simulink subsystem "VCM_main"  (R2021b)
settings: Solver=VariableStepAuto  StartTime=0.0  StopTime=10.0  RelTol=1e-3
undefined symbols (not defined in the file): df, dr, g, gear_f, gear_r, Iwf, Iwr, l, lf, M, Rwf, Rwr
libraries: simulink x47, dspstat3 x2, dspswit3 x1
(part 3 of 4)

== system VCM_main/Error display Box/Error Info3/error memory MC4 ==
  Error info : Inport
  Error triger : Inport  Port=2
  Triggered Subsystem : Subsystem  TreatAsAtomicUnit=on
  error1 : Outport  VectorParamsAs1DForOutWhenUnconnected=off
  error2 : Outport  Port=2  VectorParamsAs1DForOutWhenUnconnected=off
  error3 : Outport  Port=3  VectorParamsAs1DForOutWhenUnconnected=off
  wires:
  Triggered Subsystem/3(Out3) -> error3/1
  Error triger/1 -> Triggered Subsystem/Trigger
  Triggered Subsystem/2(Out2) -> error2/1
  Triggered Subsystem/1(Out1) -> error1/1
  Error info/1 -> Triggered Subsystem/1(In1)

== system VCM_main/VDC/80kw_limitation/Power Limit_last ==
  LimitTorque : Inport
  Power Consumption : Inport  Port=2
  Torque : Inport  Port=3
  Add : Sum  Inputs=+-
  Bus Creator : BusCreator  Inputs=4
  Bus Selector1 : BusSelector  OutputSignals=RR.torque
  Bus Selector2 : BusSelector  OutputSignals=RR,RL,FR,FL
  Bus Selector3 : BusSelector  OutputSignals=FR.torque
  Bus Selector4 : BusSelector  OutputSignals=RR.torque
  Bus Selector5 : BusSelector  OutputSignals=FL.torque
  Compare To Zero : simulink/Logic and Bit Operations/Compare To Zero  relop=<  OutDataTypeStr=boolean
  Constant : Constant  Value=80000
  Divide : Product  Inputs=**
  FeedBack : Subsystem
  FeedBack and Switch : Subsystem
  FeedBack and Switch1 : Subsystem
  FeedBack and Switch2 : Subsystem
  FeedBack and Switch3 : Subsystem
  FeedBack1 : Subsystem
  FeedBack2 : Subsystem
  FeedBack3 : Subsystem
  Gain : Gain  Gain=0
  Scope : Scope
  Scope1 : Scope
  Scope2 : Scope
  TrqOut : Outport  VectorParamsAs1DForOutWhenUnconnected=off
  wires:
  Torque/1 -> Bus Selector4/1, Bus Selector3/1, Bus Selector5/1, Bus Selector1/1
  Bus Selector5/1 -> FeedBack and Switch3/2(Torque)  "<torque>"
  Bus Selector3/1 -> FeedBack and Switch2/2(Torque)  "<torque>"
  Bus Selector1/1 -> FeedBack and Switch1/2(Torque)  "<torque>"
  FeedBack3/1(FB Torque) -> FeedBack and Switch3/1(LimitTorque)
  FeedBack2/1(FB Torque) -> FeedBack and Switch2/1(LimitTorque)
  FeedBack1/1(FB Torque) -> FeedBack and Switch1/1(LimitTorque)
  Bus Selector4/1 -> FeedBack and Switch/2(Torque)  "<torque>"
  FeedBack/1(FB Torque) -> FeedBack and Switch/1(LimitTorque)
  Divide/1 -> FeedBack2/2(FB), FeedBack1/2(FB), FeedBack/2(FB), FeedBack3/2(FB), Scope1/1
  Bus Selector2/4 -> FeedBack3/1(Torque)  "<FL>"
  Bus Selector2/3 -> FeedBack2/1(Torque)  "<FR>"
  Bus Selector2/2 -> FeedBack1/1(Torque)  "<RL>"
  FeedBack and Switch/1(trq) -> Bus Creator/1  "RRtorque"
  FeedBack and Switch3/1(trq) -> Bus Creator/4  "FLtorque"
  Bus Creator/1 -> TrqOut/1, Scope2/1
  FeedBack and Switch1/1(trq) -> Bus Creator/2  "RLtorque"
  FeedBack and Switch2/1(trq) -> Bus Creator/3  "FRtorque"
  Bus Selector2/1 -> FeedBack/1(Torque)  "<RR>"
  LimitTorque/1 -> Bus Selector2/1
  Gain/1 -> Divide/2
  Compare To Zero/1 -> Divide/1
  Add/1 -> Compare To Zero/1, Gain/1
  Power Consumption/1 -> Add/2, Scope/1
  Constant/1 -> Add/1

== system VCM_main/VDC/80kw_limitation/signal select ==
  Torque : Inport
  Bus Creator{,1..3} (4 alike) : BusCreator  Inputs=2
  Bus Creator4 : BusCreator  Inputs=4
  Bus Selector : BusSelector  OutputSignals=RR.torque,RL.torque,FR.torque,FL.torque
  Torque Speed : Outport  VectorParamsAs1DForOutWhenUnconnected=off
  wires:
  Bus Selector/4 -> Bus Creator2/1  "<torque>"
  Bus Selector/3 -> Bus Creator3/1  "<torque>"
  Bus Selector/2 -> Bus Creator1/1  "<torque>"
  Bus Selector/1 -> Bus Creator/1  "<torque>"
  [FL_ActualSpeed] -> Bus Creator2/2  "speed"
  [FR_ActualSpeed] -> Bus Creator3/2  "speed"
  [RL_ActualSpeed] -> Bus Creator1/2  "speed"
  [RR_ActualSpeed] -> Bus Creator/2  "speed"
  Bus Creator4/1 -> Torque Speed/1
  Bus Creator2/1 -> Bus Creator4/4  "FL"
  Bus Creator3/1 -> Bus Creator4/3  "FR"
  Bus Creator1/1 -> Bus Creator4/2  "RL"
  Bus Creator/1 -> Bus Creator4/1  "RR"
  Torque/1 -> Bus Selector/1

== system VCM_main/VDC/DYC1/DYC Switch ==
  Torque In : Inport
  DYC_Torque : Inport  Port=2
  Logical Operator : Logic  AllPortsSameDT=off  OutDataTypeStr=boolean
  Switch : Switch  Criteria=u2 > Threshold  Threshold=0.5
  torque : Outport
  wires:
  Logical Operator/1 -> Switch/2
  [All_bQuitInverterOn] -> Logical Operator/2
  Switch/1 -> torque/1
  [DYCOn] -> Logical Operator/1
  DYC_Torque/1 -> Switch/1  "torque"
  Torque In/1 -> Switch/3

== system VCM_main/VDC/DYC1/DYC Switch1 ==
  Torque In : Inport
  DYC_Torque : Inport  Port=2
  Logical Operator : Logic  AllPortsSameDT=off  OutDataTypeStr=boolean
  Switch : Switch  Criteria=u2 > Threshold  Threshold=0.5
  torque : Outport
  wires:
  Torque In/1 -> Switch/3
  DYC_Torque/1 -> Switch/1  "torque"
  [DYCOn] -> Logical Operator/1
  Switch/1 -> torque/1
  [All_bQuitInverterOn] -> Logical Operator/2
  Logical Operator/1 -> Switch/2

== system VCM_main/VDC/DYC1/DYC Switch2 ==
  Torque In : Inport
  DYC_Torque : Inport  Port=2
  Logical Operator : Logic  AllPortsSameDT=off  OutDataTypeStr=boolean
  Switch : Switch  Criteria=u2 > Threshold  Threshold=0.5
  torque : Outport
  wires:
  Logical Operator/1 -> Switch/2
  [All_bQuitInverterOn] -> Logical Operator/2
  Switch/1 -> torque/1
  [DYCOn] -> Logical Operator/1
  DYC_Torque/1 -> Switch/1  "torque"
  Torque In/1 -> Switch/3

== system VCM_main/VDC/DYC1/DYC Switch3 ==
  Torque In : Inport
  DYC_Torque : Inport  Port=2
  Logical Operator : Logic  AllPortsSameDT=off  OutDataTypeStr=boolean
  Switch : Switch  Criteria=u2 > Threshold  Threshold=0.5
  torque : Outport
  wires:
  Torque In/1 -> Switch/3
  DYC_Torque/1 -> Switch/1  "torque"
  [DYCOn] -> Logical Operator/1
  Switch/1 -> torque/1
  [All_bQuitInverterOn] -> Logical Operator/2
  Logical Operator/1 -> Switch/2

== system VCM_main/VDC/DYC1/DYC main ==
  Total Torque In : Inport
  DriverInput : Inport  Port=2
  Sensor : Inport  Port=3
  Bus Creator : BusCreator  Inputs=6
  Bus Creator1 : BusCreator  Inputs=6
  Bus Creator2 : BusCreator  Inputs=2
  Bus Selector : BusSelector  OutputSignals=Gain,Moment,DYCtrq_RR,DYCtrq_RL,DYCtrq_FR,DYCtrq_FL
  DYC ecopa spec : Subsystem  TreatAsAtomicUnit=on
  DYC mode1 : Subsystem  TreatAsAtomicUnit=on
  If1 : If  IfExpression=u1 == 0  ElseIfExpressions=u1<=1
  Merge : Merge
  Saturation : Saturate  UpperLimit=1  LowerLimit=0
  Terminator : Terminator
  DYC_RR : Outport
  DYC_RL : Outport  Port=2
  DYC_FR : Outport  Port=3
  DYC_FL : Outport  Port=4
  Gain : Outport  Port=5
  Moment : Outport  Port=6
  wires:
  Bus Creator2/1 -> DYC mode1/4(from_steerSW)
  [Kfb2_delta] -> Bus Creator2/2  "Kfb2_delta"
  [Km_delta] -> Bus Creator2/1  "Km_delta"
  [DYCmode] -> Saturation/1
  Bus Selector/6 -> DYC_FL/1  "<DYCtrq_FL>"
  Bus Selector/5 -> DYC_FR/1  "<DYCtrq_FR>"
  Bus Selector/4 -> DYC_RL/1  "<DYCtrq_RL>"
  Bus Selector/3 -> DYC_RR/1  "<DYCtrq_RR>"
  Bus Selector/2 -> Moment/1  "<Moment>"
  Bus Selector/1 -> Gain/1  "<Gain>"
  Merge/1 -> Bus Selector/1
  Bus Creator1/1 -> Merge/2
  Bus Creator/1 -> Merge/1
  DYC mode1/6(DYC_FL) -> Bus Creator1/6
  DYC mode1/5(DYC_FR) -> Bus Creator1/5
  DYC mode1/4(DYC_RL) -> Bus Creator1/4
  DYC mode1/3(DYC_RR) -> Bus Creator1/3
  DYC mode1/2(DYC_M) -> Bus Creator1/2  "Moment"
  DYC mode1/1(DYC_K) -> Bus Creator1/1  "Gain"
  Saturation/1 -> If1/1
  If1/3 -> Terminator/1
  If1/2 -> DYC mode1/Action
  If1/1 -> DYC ecopa spec/Action
  DYC ecopa spec/1(DYC_K) -> Bus Creator/1  "Gain"
  DYC ecopa spec/4(DYC_RL) -> Bus Creator/4
  DYC ecopa spec/5(DYC_FR) -> Bus Creator/5
  DYC ecopa spec/2(DYC_M) -> Bus Creator/2  "Moment"
  DYC ecopa spec/3(DYC_RR) -> Bus Creator/3
  DYC ecopa spec/6(DYC_FL) -> Bus Creator/6
  Total Torque In/1 -> DYC ecopa spec/1(Total Torque In), DYC mode1/1(Total Torque In)
  Sensor/1 -> DYC ecopa spec/3(Sensor), DYC mode1/3(Sensor)
  DriverInput/1 -> DYC ecopa spec/2(DriverInput), DYC mode1/2(DriverInput)

== system VCM_main/VDC/Launch/max rpm ==
  Can Inv : Inport
  Bus Selector4 : BusSelector  OutputSignals=MC_11.MC1_Actual speed value in 1/rpm,MC_31.MC3_Actual speed value in 1/rpm,MC_21.MC2_Actual speed value in 1/rpm,MC_41.MC4_Actual speed value in 1/rpm
  Min : MinMax  Function=max  Inputs=4
  max rpm : Outport
  wires:
  Bus Selector4/2 -> Min/2  "<MC3_Actual speed value in 1/rpm>"
  Bus Selector4/3 -> Min/3  "<MC2_Actual speed value in 1/rpm>"
  Bus Selector4/1 -> Min/1  "<MC1_Actual speed value in 1/rpm>"
  Min/1 -> max rpm/1  "max rpm"
  Can Inv/1 -> Bus Selector4/1
  Bus Selector4/4 -> Min/4  "<MC4_Actual speed value in 1/rpm>"

== system VCM_main/VDC/Subsystem/Subsystem ==
  note: 4コ合計
  In1 : Inport
  IVT : Inport  Port=2
  Bus Selector : BusSelector  OutputSignals=MC_11.MC1_Actual speed value in 1/rpm
  Bus Selector1 : BusSelector  OutputSignals=IVT_Msg_Result_U1
  C : Gain
  Divide : Product  Inputs=**
  Divide1 : Product  Inputs=*//
  Gain : Gain  Gain=100
  Gear : Constant  Value=13.75
  Rated Capacity(A) : Constant  Value=10
  max torque : Outport
  wires:
  Gain/1 -> Divide/2
  Bus Selector1/1 -> Gain/1  "<IVT_Msg_Result_U1>"
  Divide1/1 -> max torque/1  "max torque"
  Gear/1 -> Divide1/3
  IVT/1 -> Bus Selector1/1
  Divide/1 -> Divide1/1
  Bus Selector/1 -> Divide1/2  "<MC1_Actual speed value in 1/rpm>"
  C/1 -> Divide/1
  Rated Capacity(A)/1 -> C/1
  In1/1 -> Bus Selector/1

== system VCM_main/VDC/Subsystem1/Subsystem ==
  CAN from INV : Inport
  IVT : Inport  Port=2
  Bus Selector : BusSelector  OutputSignals=MC_11.MC1_Actual speed value in 1/rpm
  Bus Selector1 : BusSelector  OutputSignals=IVT_Msg_Result_U1
  C : Gain
  Divide : Product  Inputs=**
  Divide1 : Product  Inputs=*//
  Gain : Gain  Gain=100
  Gear : Constant  Value=13.75
  Rated Capacity(A) : Constant  Value=10
  Out1 : Outport
  wires:
  Gain/1 -> Divide/2
  Bus Selector1/1 -> Gain/1  "<IVT_Msg_Result_U1>"
  Divide1/1 -> Out1/1
  Gear/1 -> Divide1/3
  IVT/1 -> Bus Selector1/1
  Divide/1 -> Divide1/1
  Bus Selector/1 -> Divide1/2  "<MC1_Actual speed value in 1/rpm>"
  C/1 -> Divide/1
  Rated Capacity(A)/1 -> C/1
  CAN from INV/1 -> Bus Selector/1

== system VCM_main/VDC/Subsystem1/ideal brake torque for real time ==
  In1 : Inport
  Add : Sum  Inputs=-+
  Add1 : Sum
  Add2 : Sum  Inputs=-+
  Constant5 : Constant
  Divide : Product  Inputs=**
  Divide1 : Product  Inputs=***
  Divide2 : Product  Inputs=*/
  Divide3 : Product  Inputs=**
  Gain : Gain  Gain=0.2
  Gain1 : Gain  Gain=0.2
  Gain2 : Gain  Gain=1/2
  Gain3 : Gain  Gain=1/2
  hight of center of gravity : Constant  Value=0.26
  mass : Constant  Value=280
  static braking balance of front : Constant  Value=0.52
  wheel base : Constant  Value=1.53
  front ideal braking torque : Outport
  rear ideal braking torque : Outport  Port=2
  wires:
  Gain3/1 -> rear ideal braking torque/1
  Gain2/1 -> front ideal braking torque/1
  Gain/1 -> Gain2/1
  Gain1/1 -> Gain3/1
  Add2/1 -> Gain1/1  "rear ideal braking force"
  Add1/1 -> Gain/1  "front ideal braking force"
  In1/1 -> Divide1/1
  Divide/1 -> Add1/1  "front static load"
  Constant5/1 -> Add/2
  hight of center of gravity/1 -> Divide2/1
  Add/1 -> Divide3/2
  wheel base/1 -> Divide2/2
  static braking balance of front/1 -> Add/1, Divide/1
  Divide1/1 -> Add2/1, Add1/2
  Divide3/1 -> Add2/2  "rear static load"
  mass/1 -> Divide1/2, Divide/2, Divide3/1
  Divide2/1 -> Divide1/3

== system VCM_main/VDC/Torque Front//rear distributor Main/Max Torque Limit ==
  note: MAXトルクオーバーしている分だけもう一方に振り直し
  Max Torque : Inport
  torque_front : Inport  Port=2
  torque_rear : Inport  Port=3
  Add10 : Sum  Inputs=-+
  Add11 : Sum
  Add4 : Sum  Inputs=+-
  Add7 : Sum  Inputs=+-
  Add8 : Sum
  Add9 : Sum  Inputs=+-
  Display : Display
  Display5 : Display
  Display6 : Display
  Saturation : Saturate  UpperLimit=inf  LowerLimit=0
  Saturation3 : Saturate  UpperLimit=inf  LowerLimit=0
  torque_front Out : Outport
  torque_rear Out : Outport  Port=2
  wires:
  Max Torque/1 -> Add9/2, Add4/2
  Add11/1 -> torque_rear Out/1
  Add7/1 -> Add11/2
  Add4/1 -> Saturation/1
  Add10/1 -> torque_front Out/1
  Add8/1 -> Add10/2
  torque_rear/1 -> Display6/1, Add7/1, Add4/1
  Add9/1 -> Saturation3/1
  torque_front/1 -> Display5/1, Add8/1, Add9/1
  Saturation3/1 -> Add10/1, Add11/1
  Saturation/1 -> Display/1, Add7/2, Add8/2

== system VCM_main/VDC/Torque Front//rear distributor Main/Min Torque Limit ==
  note: MINトルクオーバーしている分だけもう一方に振り直し
  Min Torque : Inport
  torque_front : Inport  Port=2
  torque_rear : Inport  Port=3
  Add10 : Sum  Inputs=-+
  Add11 : Sum
  Add4 : Sum  Inputs=+-
  Add7 : Sum  Inputs=+-
  Add8 : Sum
  Add9 : Sum  Inputs=+-
  Display{,1..2,5..6} (5 alike) : Display
  Gain : Gain  Gain=-1
  Saturation : Saturate  UpperLimit=0  LowerLimit=-inf
  Saturation3 : Saturate  UpperLimit=0  LowerLimit=-inf
  torque_rear Out : Outport
  torque_front Out : Outport  Port=2
  wires:
  Gain/1 -> Add9/2, Add4/2
  Min Torque/1 -> Gain/1
  Add11/1 -> torque_rear Out/1  "torque_rear"
  Add7/1 -> Add11/2, Display1/1
  Add4/1 -> Saturation/1
  Add10/1 -> torque_front Out/1  "torque_front"
  Add8/1 -> Add10/2
  torque_rear/1 -> Display6/1, Add7/1, Add4/1
  Add9/1 -> Saturation3/1
  torque_front/1 -> Display5/1, Add8/1, Add9/1
  Saturation3/1 -> Add10/1, Add11/1, Display2/1
  Saturation/1 -> Display/1, Add7/2, Add8/2

== system VCM_main/VDC/Torque Front//rear distributor Main/Saturation ==
  u : Inport
  Saturation Dynamic1 : simulink/Discontinuities/Saturation Dynamic  OutMin=[]  OutMax=[]  OutDataTypeStr=Inherit: Same as second input  OutDataType=fixdt(1, 16)  OutScaling=2^-10  DoSatur=off
  y : Outport
  wires:
  [MinTorque] -> Saturation Dynamic1/3
  u/1 -> Saturation Dynamic1/2
  Saturation Dynamic1/1 -> y/1
  [MaxTorque] -> Saturation Dynamic1/1

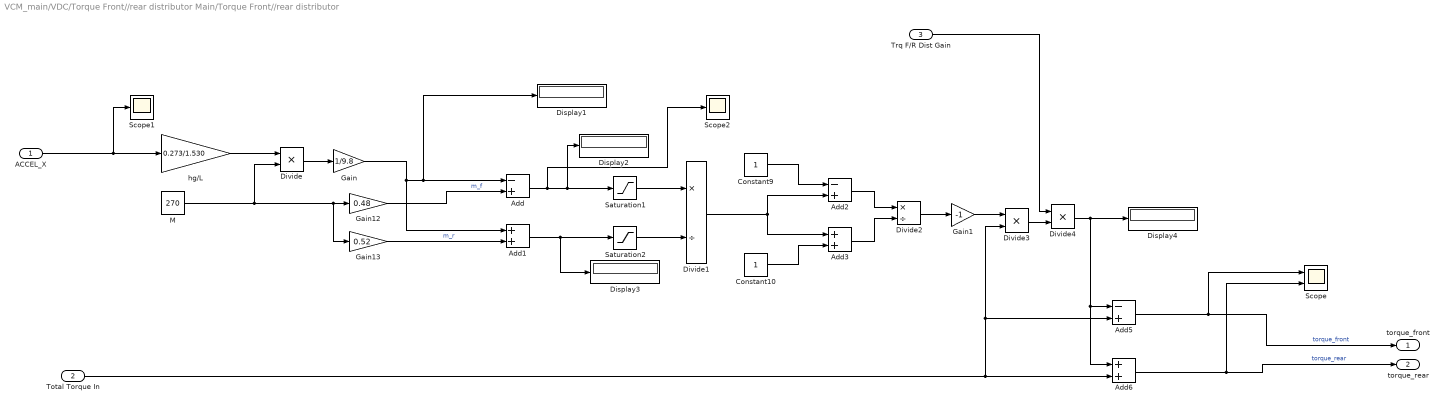
== system VCM_main/VDC/Torque Front//rear distributor Main/Torque Front//rear distributor  ==
  ACCEL_X : Inport
  Total Torque In : Inport  Port=2
  Trq F/R Dist Gain : Inport  Port=3
  Add : Sum  Inputs=-+
  Add1 : Sum
  Add2 : Sum  Inputs=-+
  Add3 : Sum
  Add5 : Sum  Inputs=-+
  Add6 : Sum
  Constant10 : Constant
  Constant9 : Constant
  Display{1..4} (4 alike) : Display
  Divide : Product  Inputs=**
  Divide1 : Product  Inputs=*/
  Divide2 : Product  Inputs=*/
  Divide3 : Product  Inputs=**
  Divide4 : Product  Inputs=**
  Gain : Gain  Gain=1/9.8
  Gain1 : Gain  Gain=-1
  Gain12 : Gain  Gain=0.48
  Gain13 : Gain  Gain=0.52
  M : Constant  Value=270
  Saturation1 : Saturate  UpperLimit=270  LowerLimit=10
  Saturation2 : Saturate  UpperLimit=270  LowerLimit=10
  Scope : Scope  NumInputPorts=2
  Scope1 : Scope
  Scope2 : Scope
  hg/L : Gain  Gain=0.273/1.530
  torque_front : Outport
  torque_rear : Outport  Port=2
  wires:
  Divide/1 -> Gain/1
  Total Torque In/1 -> Divide3/2, Add5/2, Add6/2
  Trq F/R Dist Gain/1 -> Divide4/1
  Divide3/1 -> Divide4/2
  Add5/1 -> torque_front/1, Scope/1  "torque_front"
  Add6/1 -> torque_rear/1, Scope/2  "torque_rear"
  Gain13/1 -> Add1/2  "m_r"
  Saturation1/1 -> Divide1/1
  Add/1 -> Saturation1/1, Display2/1, Scope2/1
  Gain/1 -> Add/1, Display1/1, Add1/1
  Add1/1 -> Saturation2/1, Display3/1
  ACCEL_X/1 -> hg/L/1, Scope1/1
  hg/L/1 -> Divide/1
  Constant10/1 -> Add3/2
  Gain1/1 -> Divide3/1
  Add2/1 -> Divide2/1
  Gain12/1 -> Add/2  "m_f"
  Divide2/1 -> Gain1/1
  Constant9/1 -> Add2/1
  Saturation2/1 -> Divide1/2
  Divide4/1 -> Display4/1, Add5/1, Add6/1
  Add3/1 -> Divide2/2
  Divide1/1 -> Add2/2, Add3/1
  M/1 -> Gain12/1, Gain13/1, Divide/2

== system VCM_main/VDC/Traction Control/Acc Estimater ==
  1/Gear{1..4} (4 alike) : Gain  Gain=gear_r
  Add : Sum  Inputs=++++
  EstLongAcc1 : Scope
  Gain : Gain  Gain=1/(M+2*Iwf/Rwf/Rwf+2*Iwr/Rwr/Rwr)
  Gain1 : Gain  Gain=1/g
  Moving Average : dspstat3/Moving Average  Method=Sliding window  ForgettingFactorPort=off  SpecifyWindowLength=on  WindowLength=10  ForgettingFactor=0.9  SimulateUsing=Code generation
  Rtire{1..4} (4 alike) : Gain  Gain=1/Rwf
  Saturation : Saturate  UpperLimit=1.3*g  LowerLimit=-1.3*g
  EstLongAcc : Outport
  wires:
  [FL_Torque] -> 1/Gear2/1
  Gain/1 -> Moving Average/1  "LongAcc"
  Rtire1/1 -> Add/1
  [RL_Torque] -> 1/Gear4/1
  Rtire3/1 -> Add/3
  1/Gear3/1 -> Rtire4/1
  [FR_Torque] -> 1/Gear1/1
  1/Gear2/1 -> Rtire1/1
  Saturation/1 -> EstLongAcc/1, Gain1/1  "LongAcc"
  Rtire2/1 -> Add/2
  Add/1 -> Gain/1
  1/Gear1/1 -> Rtire2/1
  Gain1/1 -> EstLongAcc1/1
  Rtire4/1 -> Add/4
  1/Gear4/1 -> Rtire3/1
  Moving Average/1 -> Saturation/1
  [RR_Torque] -> 1/Gear3/1

== system VCM_main/VDC/Traction Control/ActualSpeed ==
  Bus Creator : BusCreator  Inputs=4
  ActualSpeed : Outport
  wires:
  [RL_ActualSpeed] -> Bus Creator/3  "RL"
  [FR_ActualSpeed] -> Bus Creator/2  "FR"
  [FL_ActualSpeed] -> Bus Creator/1  "FL"
  [RR_ActualSpeed] -> Bus Creator/4  "RR"
  Bus Creator/1 -> ActualSpeed/1  "ActualSpeed"

== system VCM_main/VDC/Traction Control/Fx Estimater ==
  Bus Creator : BusCreator  Inputs=4
  EstFx : Scope
  FxEstimater : Subsystem
  FxEstimater1 : Subsystem
  FxEstimater2 : Subsystem
  FxEstimater3 : Subsystem
  Fx : Outport
  wires:
  FxEstimater1/1(Fx) -> Bus Creator/2  "FR"
  Bus Creator/1 -> Fx/1, EstFx/1  "Fx"
  FxEstimater3/1(Fx) -> Bus Creator/4  "RR"
  FxEstimater2/1(Fx) -> Bus Creator/3  "RL"
  FxEstimater/1(Fx) -> Bus Creator/1  "FL"
  [FL_Torque] -> FxEstimater/1(Torque)
  [FL_ActualSpeed] -> FxEstimater/2(ActualSpeed)
  [FR_ActualSpeed] -> FxEstimater1/2(ActualSpeed)
  [FR_Torque] -> FxEstimater1/1(Torque)
  [RR_Torque] -> FxEstimater3/1(Torque)
  [RR_ActualSpeed] -> FxEstimater3/2(ActualSpeed)
  [RL_ActualSpeed] -> FxEstimater2/2(ActualSpeed)
  [RL_Torque] -> FxEstimater2/1(Torque)

== system VCM_main/VDC/Traction Control/Load Estimater ==
  Long Acc : Inport
  Sensor : Inport  Port=2
  Steer : Inport  Port=3
  Bus Creator : BusCreator  Inputs=4
  Bus Selector : BusSelector  OutputSignals=CAN_from_IMU_139.VELOCITY_X
  Bus Selector1 : BusSelector  OutputSignals=CAN_from_IMU_121.ACCEL_Y
  Constant : Constant  Value=l
  Divide : Product  Inputs=*/
  Divide1 : Product  Inputs=*/
  EstAcc : Scope  NumInputPorts=2
  EstLoad : Scope
  FR Load Diff : Subsystem  ReferencedSubsystem=FR_Load_Diff
  Gain : Gain  Gain=1/(2*pi)
  Off : Gain  Gain=0
  Product : Product
  RL Load Diff : Subsystem  ReferencedSubsystem=RL_Load_Diff
  Load : Outport
  wires:
  Constant/1 -> Divide/1
  Divide/1 -> Divide1/2  "R"
  RL Load Diff/4 -> Bus Creator/4  "RR"
  Divide1/1 -> EstAcc/2
  Steer/1 -> Gain/1
  RL Load Diff/1 -> Bus Creator/1  "FL"
  FR Load Diff/1 -> RL Load Diff/1  "FrontLoad"
  Bus Selector1/1 -> Off/1  "<ACCEL_Y>"
  FR Load Diff/2 -> RL Load Diff/2  "RearLoad"
  RL Load Diff/2 -> Bus Creator/2  "FR"
  Long Acc/1 -> FR Load Diff/1, EstAcc/1
  RL Load Diff/3 -> Bus Creator/3  "RL"
  Gain/1 -> Divide/2
  Off/1 -> RL Load Diff/3
  Bus Creator/1 -> Load/1, EstLoad/1  "Load"
  Sensor/1 -> Bus Selector1/1, Bus Selector/1
  Bus Selector/1 -> Product/1, Product/2  "<VELOCITY_X>"
  Product/1 -> Divide1/1

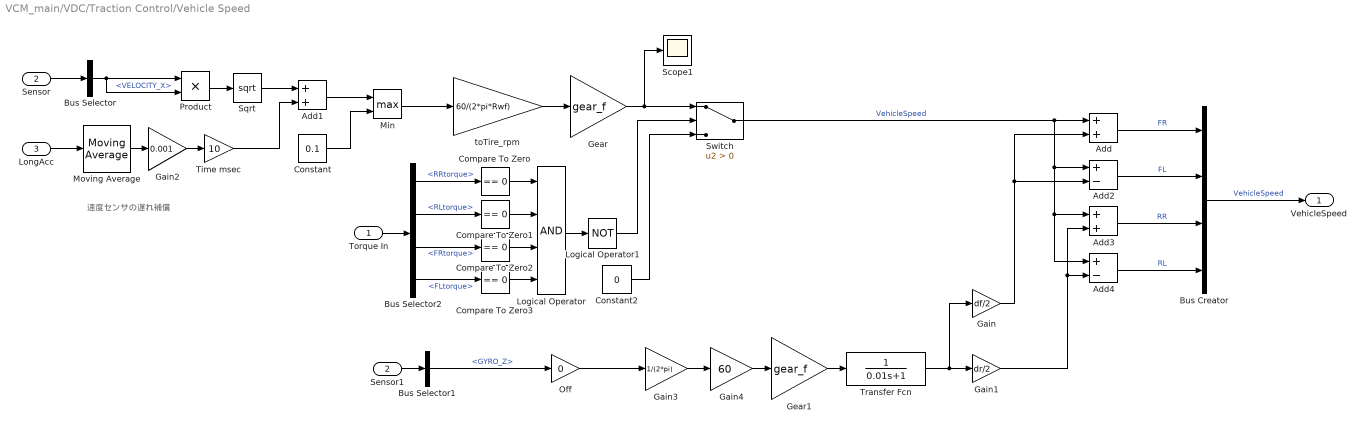
== system VCM_main/VDC/Traction Control/Vehicle Speed ==
  note: 速度センサの遅れ補償
  Torque In : Inport
  Sensor : Inport  Port=2
  LongAcc : Inport  Port=3
  Add : Sum
  Add1 : Sum
  Add2 : Sum  Inputs=+-
  Add3 : Sum
  Add4 : Sum  Inputs=+-
  Bus Creator : BusCreator  Inputs=4
  Bus Selector : BusSelector  OutputSignals=CAN_from_IMU_139.VELOCITY_X
  Bus Selector1 : BusSelector  OutputSignals=CAN_from_IMU_122.GYRO_Z
  Bus Selector2 : BusSelector  OutputSignals=RRtorque,RLtorque,FRtorque,FLtorque
  Compare To Zero{,1..3} (4 alike) : simulink/Logic and Bit Operations/Compare To Zero  relop===  OutDataTypeStr=boolean
  Constant : Constant  Value=0.1
  Constant2 : Constant  Value=0
  Gain : Gain  Gain=df/2
  Gain1 : Gain  Gain=dr/2
  Gain2 : Gain  Gain=0.001
  Gain3 : Gain  Gain=1/(2*pi)
  Gain4 : Gain  Gain=60
  Gear : Gain  Gain=gear_f
  Gear1 : Gain  Gain=gear_f
  Logical Operator : Logic  Inputs=4  AllPortsSameDT=off  OutDataTypeStr=boolean
  Logical Operator1 : Logic  Operator=NOT  AllPortsSameDT=off  OutDataTypeStr=boolean
  Min : MinMax  Function=max  Inputs=2
  Moving Average : dspstat3/Moving Average  Method=Sliding window  ForgettingFactorPort=off  SpecifyWindowLength=on  WindowLength=80  ForgettingFactor=0.9  SimulateUsing=Code generation
  Off : Gain  Gain=0
  Product : Product
  Scope1 : Scope
  Sensor1 : InportShadow  Port=2
  Sqrt : Sqrt  SaturateOnIntegerOverflow=on
  Switch : Switch  Criteria=u2 > Threshold
  Time msec : Gain  Gain=10
  Transfer Fcn : TransferFcn  Denominator=[0.01 1]
  toTire_rpm : Gain  Gain=60/(2*pi*Rwf)
  VehicleSpeed : Outport
  wires:
  Gain3/1 -> Gain4/1
  Bus Selector1/1 -> Off/1  "<GYRO_Z>"
  Product/1 -> Sqrt/1
  Transfer Fcn/1 -> Gain1/1, Gain/1
  Bus Selector/1 -> Product/1, Product/2  "<VELOCITY_X>"
  Switch/1 -> Add/1, Add2/1, Add4/1, Add3/1  "VehicleSpeed"
  Compare To Zero/1 -> Logical Operator/1
  Sensor/1 -> Bus Selector/1
  Bus Selector2/4 -> Compare To Zero3/1  "<FLtorque>"
  Compare To Zero2/1 -> Logical Operator/3
  Torque In/1 -> Bus Selector2/1
  LongAcc/1 -> Moving Average/1
  Sqrt/1 -> Add1/1
  Gear/1 -> Scope1/1, Switch/1
  toTire_rpm/1 -> Gear/1
  Gain1/1 -> Add3/2, Add4/2
  Logical Operator/1 -> Logical Operator1/1
  Add3/1 -> Bus Creator/3  "RR"
  Bus Selector2/1 -> Compare To Zero/1  "<RRtorque>"
  Logical Operator1/1 -> Switch/2
  Sensor1/1 -> Bus Selector1/1
  Compare To Zero3/1 -> Logical Operator/4
  Constant/1 -> Min/2
  Bus Selector2/2 -> Compare To Zero1/1  "<RLtorque>"
  Time msec/1 -> Add1/2
  Bus Selector2/3 -> Compare To Zero2/1  "<FRtorque>"
  Compare To Zero1/1 -> Logical Operator/2
  Off/1 -> Gain3/1
  Constant2/1 -> Switch/3
  Min/1 -> toTire_rpm/1
  Gain/1 -> Add/2, Add2/2
  Add1/1 -> Min/1
  Add2/1 -> Bus Creator/2  "FL"
  Moving Average/1 -> Gain2/1
  Add/1 -> Bus Creator/1  "FR"
  Add4/1 -> Bus Creator/4  "RL"
  Gain2/1 -> Time msec/1
  Gain4/1 -> Gear1/1
  Bus Creator/1 -> VehicleSpeed/1  "VehicleSpeed"
  Gear1/1 -> Transfer Fcn/1

== system VCM_main/VDC/VCM_Status/Sliprate ==
  from Sensor : Inport
  Bus Creator : BusCreator  Inputs=4
  Bus Selector4 : BusSelector  OutputSignals=CAN_from_IMU_139.VELOCITY_X
  Scope : Scope  NumInputPorts=4
  SlipRateClc FL : Subsystem  ReferencedSubsystem=SlipRateClc
  SlipRateClc FR : Subsystem  ReferencedSubsystem=SlipRateClc
  SlipRateClc RL : Subsystem  ReferencedSubsystem=SlipRateClc
  SlipRateClc RR : Subsystem  ReferencedSubsystem=SlipRateClc
  Tire rpm{,1..3} (4 alike) : Gain  Gain=1/gear_f
  to m/s{,1..3} (4 alike) : Gain  Gain=(2*pi*Rwf)/60
  Sliprate : Outport
  wires:
  to m/s1/1 -> SlipRateClc RR/1
  Tire rpm3/1 -> to m/s3/1
  SlipRateClc FR/1 -> Bus Creator/4, Scope/4  "FR"
  Bus Selector4/1 -> SlipRateClc FR/2, SlipRateClc RL/2, SlipRateClc RR/2, SlipRateClc FL/2  "<VELOCITY_X>"
  SlipRateClc RR/1 -> Bus Creator/2, Scope/2  "RR"
  SlipRateClc FL/1 -> Bus Creator/1, Scope/1  "FL"
  Bus Creator/1 -> Sliprate/1  "Sliprate"
  SlipRateClc RL/1 -> Bus Creator/3, Scope/3  "RL"
  Tire rpm1/1 -> to m/s1/1
  to m/s/1 -> SlipRateClc FL/1
  [FL_ActualSpeed] -> Tire rpm/1
  to m/s2/1 -> SlipRateClc RL/1
  Tire rpm/1 -> to m/s/1
  [RL_ActualSpeed] -> Tire rpm2/1
  [FR_ActualSpeed] -> Tire rpm3/1
  [RR_ActualSpeed] -> Tire rpm1/1
  to m/s3/1 -> SlipRateClc FR/1
  Tire rpm2/1 -> to m/s2/1
  from Sensor/1 -> Bus Selector4/1

== system VCM_main/VDC/VCM_Status/VCMStatus_bus ==
  In1 : Inport
  Bus Creator1 : BusCreator  Inputs=7
  Logical Operator1 : Logic  AllPortsSameDT=off  OutDataTypeStr=boolean
  VCMStatus : Outport
  wires:
  Bus Creator1/1 -> VCMStatus/1  "VCMStatus"
  In1/1 -> Logical Operator1/1
  [PowerLimitOn] -> Bus Creator1/7  "80kWOn"
  [TCOn] -> Bus Creator1/4  "TCOn"
  Logical Operator1/1 -> Bus Creator1/1  "VDCStatus"
  [VDCOn] -> Logical Operator1/2
  [DYCOn] -> Bus Creator1/6  "DYCOn"
  [ABSOn] -> Bus Creator1/5  "ABSOn"
  [BrakeOverRide] -> Bus Creator1/3  "BrakeOverRide"
  [APPS_SafetyError] -> Bus Creator1/2  "APPS_SafetyError"

== system VCM_main/Error display Box/Error Info/error memory MC1/Triggered Subsystem ==
  In1 : Inport
  Trigger : TriggerPort  VariantControl=Variant
  Delay : Delay  DelayLength=1  InitialCondition=0
  Delay1 : Delay  InitialCondition=0
  Out1 : Outport  VectorParamsAs1DForOutWhenUnconnected=off
  Out2 : Outport  Port=2  InitialOutput=[0]  VectorParamsAs1DForOutWhenUnconnected=off
  Out3 : Outport  Port=3  InitialOutput=[0]  VectorParamsAs1DForOutWhenUnconnected=off
  wires:
  Delay1/1 -> Out3/1
  Delay/1 -> Out2/1
  In1/1 -> Out1/1, Delay1/1, Delay/1

== system VCM_main/Error display Box/Error Info/error memory MC2/Triggered Subsystem ==
  In1 : Inport
  Trigger : TriggerPort  VariantControl=Variant
  Delay : Delay  DelayLength=1  InitialCondition=0
  Delay1 : Delay  InitialCondition=0
  Out1 : Outport  VectorParamsAs1DForOutWhenUnconnected=off
  Out2 : Outport  Port=2  InitialOutput=[0]  VectorParamsAs1DForOutWhenUnconnected=off
  Out3 : Outport  Port=3  InitialOutput=[0]  VectorParamsAs1DForOutWhenUnconnected=off
  wires:
  Delay1/1 -> Out3/1
  Delay/1 -> Out2/1
  In1/1 -> Out1/1, Delay1/1, Delay/1

== system VCM_main/Error display Box/Error Info/error memory MC3/Triggered Subsystem ==
  In1 : Inport
  Trigger : TriggerPort  VariantControl=Variant
  Delay : Delay  DelayLength=1  InitialCondition=0
  Delay1 : Delay  InitialCondition=0
  Out1 : Outport  VectorParamsAs1DForOutWhenUnconnected=off
  Out2 : Outport  Port=2  InitialOutput=[0]  VectorParamsAs1DForOutWhenUnconnected=off
  Out3 : Outport  Port=3  InitialOutput=[0]  VectorParamsAs1DForOutWhenUnconnected=off
  wires:
  Delay1/1 -> Out3/1
  Delay/1 -> Out2/1
  In1/1 -> Out1/1, Delay1/1, Delay/1

== system VCM_main/Error display Box/Error Info/error memory MC4/Triggered Subsystem ==
  In1 : Inport
  Trigger : TriggerPort  VariantControl=Variant
  Delay : Delay  DelayLength=1  InitialCondition=0
  Delay1 : Delay  InitialCondition=0
  Out1 : Outport  VectorParamsAs1DForOutWhenUnconnected=off
  Out2 : Outport  Port=2  InitialOutput=[0]  VectorParamsAs1DForOutWhenUnconnected=off
  Out3 : Outport  Port=3  InitialOutput=[0]  VectorParamsAs1DForOutWhenUnconnected=off
  wires:
  Delay1/1 -> Out3/1
  Delay/1 -> Out2/1
  In1/1 -> Out1/1, Delay1/1, Delay/1

== system VCM_main/Error display Box/Error Info1/error memory MC1/Triggered Subsystem ==
  In1 : Inport
  Trigger : TriggerPort  VariantControl=Variant
  Delay : Delay  DelayLength=1  InitialCondition=0
  Delay1 : Delay  InitialCondition=0
  Out1 : Outport  VectorParamsAs1DForOutWhenUnconnected=off
  Out2 : Outport  Port=2  InitialOutput=[0]  VectorParamsAs1DForOutWhenUnconnected=off
  Out3 : Outport  Port=3  InitialOutput=[0]  VectorParamsAs1DForOutWhenUnconnected=off
  wires:
  Delay1/1 -> Out3/1
  Delay/1 -> Out2/1
  In1/1 -> Out1/1, Delay/1, Delay1/1

== system VCM_main/Error display Box/Error Info1/error memory MC2/Triggered Subsystem ==
  In1 : Inport
  Trigger : TriggerPort  VariantControl=Variant
  Delay : Delay  DelayLength=1  InitialCondition=0
  Delay1 : Delay  InitialCondition=0
  Out1 : Outport  VectorParamsAs1DForOutWhenUnconnected=off
  Out2 : Outport  Port=2  InitialOutput=[0]  VectorParamsAs1DForOutWhenUnconnected=off
  Out3 : Outport  Port=3  InitialOutput=[0]  VectorParamsAs1DForOutWhenUnconnected=off
  wires:
  Delay1/1 -> Out3/1
  Delay/1 -> Out2/1
  In1/1 -> Out1/1, Delay/1, Delay1/1

== system VCM_main/Error display Box/Error Info1/error memory MC3/Triggered Subsystem ==
  In1 : Inport
  Trigger : TriggerPort  VariantControl=Variant
  Delay : Delay  DelayLength=1  InitialCondition=0
  Delay1 : Delay  InitialCondition=0
  Out1 : Outport  VectorParamsAs1DForOutWhenUnconnected=off
  Out2 : Outport  Port=2  InitialOutput=[0]  VectorParamsAs1DForOutWhenUnconnected=off
  Out3 : Outport  Port=3  InitialOutput=[0]  VectorParamsAs1DForOutWhenUnconnected=off
  wires:
  Delay1/1 -> Out3/1
  Delay/1 -> Out2/1
  In1/1 -> Out1/1, Delay/1, Delay1/1

== system VCM_main/Error display Box/Error Info1/error memory MC4/Triggered Subsystem ==
  In1 : Inport
  Trigger : TriggerPort  VariantControl=Variant
  Delay : Delay  DelayLength=1  InitialCondition=0
  Delay1 : Delay  InitialCondition=0
  Out1 : Outport  VectorParamsAs1DForOutWhenUnconnected=off
  Out2 : Outport  Port=2  InitialOutput=[0]  VectorParamsAs1DForOutWhenUnconnected=off
  Out3 : Outport  Port=3  InitialOutput=[0]  VectorParamsAs1DForOutWhenUnconnected=off
  wires:
  Delay1/1 -> Out3/1
  Delay/1 -> Out2/1
  In1/1 -> Out1/1, Delay/1, Delay1/1

== system VCM_main/Error display Box/Error Info2/error memory MC1/Triggered Subsystem ==
  In1 : Inport
  Trigger : TriggerPort  VariantControl=Variant
  Delay : Delay  DelayLength=1  InitialCondition=0
  Delay1 : Delay  InitialCondition=0
  Out1 : Outport  VectorParamsAs1DForOutWhenUnconnected=off
  Out2 : Outport  Port=2  InitialOutput=[0]  VectorParamsAs1DForOutWhenUnconnected=off
  Out3 : Outport  Port=3  InitialOutput=[0]  VectorParamsAs1DForOutWhenUnconnected=off
  wires:
  Delay1/1 -> Out3/1
  Delay/1 -> Out2/1
  In1/1 -> Out1/1, Delay/1, Delay1/1

== system VCM_main/Error display Box/Error Info2/error memory MC2/Triggered Subsystem ==
  In1 : Inport
  Trigger : TriggerPort  VariantControl=Variant
  Delay : Delay  DelayLength=1  InitialCondition=0
  Delay1 : Delay  InitialCondition=0
  Out1 : Outport  VectorParamsAs1DForOutWhenUnconnected=off
  Out2 : Outport  Port=2  InitialOutput=[0]  VectorParamsAs1DForOutWhenUnconnected=off
  Out3 : Outport  Port=3  InitialOutput=[0]  VectorParamsAs1DForOutWhenUnconnected=off
  wires:
  Delay1/1 -> Out3/1
  Delay/1 -> Out2/1
  In1/1 -> Out1/1, Delay/1, Delay1/1

== system VCM_main/Error display Box/Error Info2/error memory MC3/Triggered Subsystem ==
  In1 : Inport
  Trigger : TriggerPort  VariantControl=Variant
  Delay : Delay  DelayLength=1  InitialCondition=0
  Delay1 : Delay  InitialCondition=0
  Out1 : Outport  VectorParamsAs1DForOutWhenUnconnected=off
  Out2 : Outport  Port=2  InitialOutput=[0]  VectorParamsAs1DForOutWhenUnconnected=off
  Out3 : Outport  Port=3  InitialOutput=[0]  VectorParamsAs1DForOutWhenUnconnected=off
  wires:
  Delay1/1 -> Out3/1
  Delay/1 -> Out2/1
  In1/1 -> Out1/1, Delay/1, Delay1/1

== system VCM_main/Error display Box/Error Info2/error memory MC4/Triggered Subsystem ==
  In1 : Inport
  Trigger : TriggerPort  VariantControl=Variant
  Delay : Delay  DelayLength=1  InitialCondition=0
  Delay1 : Delay  InitialCondition=0
  Out1 : Outport  VectorParamsAs1DForOutWhenUnconnected=off
  Out2 : Outport  Port=2  InitialOutput=[0]  VectorParamsAs1DForOutWhenUnconnected=off
  Out3 : Outport  Port=3  InitialOutput=[0]  VectorParamsAs1DForOutWhenUnconnected=off
  wires:
  Delay1/1 -> Out3/1
  Delay/1 -> Out2/1
  In1/1 -> Out1/1, Delay/1, Delay1/1

== system VCM_main/Error display Box/Error Info3/error memory MC1/Triggered Subsystem ==
  In1 : Inport
  Trigger : TriggerPort  VariantControl=Variant
  Delay : Delay  DelayLength=1  InitialCondition=0
  Delay1 : Delay  InitialCondition=0
  Out1 : Outport  VectorParamsAs1DForOutWhenUnconnected=off
  Out2 : Outport  Port=2  InitialOutput=[0]  VectorParamsAs1DForOutWhenUnconnected=off
  Out3 : Outport  Port=3  InitialOutput=[0]  VectorParamsAs1DForOutWhenUnconnected=off
  wires:
  Delay1/1 -> Out3/1
  Delay/1 -> Out2/1
  In1/1 -> Out1/1, Delay/1, Delay1/1

== system VCM_main/Error display Box/Error Info3/error memory MC2/Triggered Subsystem ==
  In1 : Inport
  Trigger : TriggerPort  VariantControl=Variant
  Delay : Delay  DelayLength=1  InitialCondition=0
  Delay1 : Delay  InitialCondition=0
  Out1 : Outport  VectorParamsAs1DForOutWhenUnconnected=off
  Out2 : Outport  Port=2  InitialOutput=[0]  VectorParamsAs1DForOutWhenUnconnected=off
  Out3 : Outport  Port=3  InitialOutput=[0]  VectorParamsAs1DForOutWhenUnconnected=off
  wires:
  Delay1/1 -> Out3/1
  Delay/1 -> Out2/1
  In1/1 -> Out1/1, Delay/1, Delay1/1

== system VCM_main/Error display Box/Error Info3/error memory MC3/Triggered Subsystem ==
  In1 : Inport
  Trigger : TriggerPort  VariantControl=Variant
  Delay : Delay  DelayLength=1  InitialCondition=0
  Delay1 : Delay  InitialCondition=0
  Out1 : Outport  VectorParamsAs1DForOutWhenUnconnected=off
  Out2 : Outport  Port=2  InitialOutput=[0]  VectorParamsAs1DForOutWhenUnconnected=off
  Out3 : Outport  Port=3  InitialOutput=[0]  VectorParamsAs1DForOutWhenUnconnected=off
  wires:
  Delay1/1 -> Out3/1
  Delay/1 -> Out2/1
  In1/1 -> Out1/1, Delay/1, Delay1/1

== system VCM_main/Error display Box/Error Info3/error memory MC4/Triggered Subsystem ==
  In1 : Inport
  Trigger : TriggerPort  VariantControl=Variant
  Delay : Delay  DelayLength=1  InitialCondition=0
  Delay1 : Delay  InitialCondition=0
  Out1 : Outport  VectorParamsAs1DForOutWhenUnconnected=off
  Out2 : Outport  Port=2  InitialOutput=[0]  VectorParamsAs1DForOutWhenUnconnected=off
  Out3 : Outport  Port=3  InitialOutput=[0]  VectorParamsAs1DForOutWhenUnconnected=off
  wires:
  Delay1/1 -> Out3/1
  Delay/1 -> Out2/1
  In1/1 -> Out1/1, Delay/1, Delay1/1

== system VCM_main/VDC/80kw_limitation/Power Limit_last/FeedBack ==
  Torque : Inport
  FB : Inport  Port=2
  Add : Sum
  Bus Selector3 : BusSelector  OutputSignals=torque
  FB Torque : Outport
  wires:
  Torque/1 -> Bus Selector3/1
  Add/1 -> FB Torque/1
  FB/1 -> Add/2
  Bus Selector3/1 -> Add/1  "<torque>"

== system VCM_main/VDC/80kw_limitation/Power Limit_last/FeedBack and Switch ==
  LimitTorque : Inport
  Torque : Inport  Port=2
  Max : MinMax  Function=max  Inputs=2
  Min : MinMax  Inputs=2
  Saturation Dynamic : simulink/Discontinuities/Saturation Dynamic  OutMin=[]  OutMax=[]  OutDataTypeStr=Inherit: Same as second input  OutDataType=fixdt(1, 16)  OutScaling=2^-10  DoSatur=off
  Switch : Switch  Criteria=u2 > Threshold
  Switch1 : Switch  Criteria=u2 > Threshold
  trq : Outport
  wires:
  [MinTorque] -> Saturation Dynamic/3
  Saturation Dynamic/1 -> trq/1
  Switch1/1 -> Saturation Dynamic/1  "torque"
  [PowerLimitOn] -> Switch1/2
  Switch/1 -> Switch1/1  "torque"
  Min/1 -> Switch/1
  Max/1 -> Switch/3
  Torque/1 -> Min/1, Switch/2, Max/2, Switch1/3, Saturation Dynamic/2
  LimitTorque/1 -> Min/2, Max/1

== system VCM_main/VDC/80kw_limitation/Power Limit_last/FeedBack and Switch1 ==
  LimitTorque : Inport
  Torque : Inport  Port=2
  Max : MinMax  Function=max  Inputs=2
  Min : MinMax  Inputs=2
  Saturation Dynamic : simulink/Discontinuities/Saturation Dynamic  OutMin=[]  OutMax=[]  OutDataTypeStr=Inherit: Same as second input  OutDataType=fixdt(1, 16)  OutScaling=2^-10  DoSatur=off
  Switch : Switch  Criteria=u2 > Threshold
  Switch1 : Switch  Criteria=u2 > Threshold
  trq : Outport
  wires:
  LimitTorque/1 -> Max/1, Min/2
  Torque/1 -> Saturation Dynamic/2, Switch1/3, Max/2, Switch/2, Min/1
  Max/1 -> Switch/3
  Min/1 -> Switch/1
  Switch/1 -> Switch1/1  "torque"
  [PowerLimitOn] -> Switch1/2
  Switch1/1 -> Saturation Dynamic/1  "torque"
  Saturation Dynamic/1 -> trq/1
  [MinTorque] -> Saturation Dynamic/3

== system VCM_main/VDC/80kw_limitation/Power Limit_last/FeedBack and Switch2 ==
  LimitTorque : Inport
  Torque : Inport  Port=2
  Max : MinMax  Function=max  Inputs=2
  Min : MinMax  Inputs=2
  Saturation Dynamic : simulink/Discontinuities/Saturation Dynamic  OutMin=[]  OutMax=[]  OutDataTypeStr=Inherit: Same as second input  OutDataType=fixdt(1, 16)  OutScaling=2^-10  DoSatur=off
  Switch : Switch  Criteria=u2 > Threshold
  Switch1 : Switch  Criteria=u2 > Threshold
  trq : Outport
  wires:
  [MinTorque] -> Saturation Dynamic/3
  Saturation Dynamic/1 -> trq/1
  Switch1/1 -> Saturation Dynamic/1  "torque"
  [PowerLimitOn] -> Switch1/2
  Switch/1 -> Switch1/1  "torque"
  Min/1 -> Switch/1
  Max/1 -> Switch/3
  Torque/1 -> Min/1, Switch/2, Max/2, Switch1/3, Saturation Dynamic/2
  LimitTorque/1 -> Min/2, Max/1

== system VCM_main/VDC/80kw_limitation/Power Limit_last/FeedBack and Switch3 ==
  LimitTorque : Inport
  Torque : Inport  Port=2
  Max : MinMax  Function=max  Inputs=2
  Min : MinMax  Inputs=2
  Saturation Dynamic : simulink/Discontinuities/Saturation Dynamic  OutMin=[]  OutMax=[]  OutDataTypeStr=Inherit: Same as second input  OutDataType=fixdt(1, 16)  OutScaling=2^-10  DoSatur=off
  Switch : Switch  Criteria=u2 > Threshold
  Switch1 : Switch  Criteria=u2 > Threshold
  trq : Outport
  wires:
  LimitTorque/1 -> Max/1, Min/2
  Torque/1 -> Saturation Dynamic/2, Switch1/3, Max/2, Switch/2, Min/1
  Max/1 -> Switch/3
  Min/1 -> Switch/1
  Switch/1 -> Switch1/1  "torque"
  [PowerLimitOn] -> Switch1/2
  Switch1/1 -> Saturation Dynamic/1  "torque"
  Saturation Dynamic/1 -> trq/1
  [MinTorque] -> Saturation Dynamic/3

== system VCM_main/VDC/80kw_limitation/Power Limit_last/FeedBack1 ==
  Torque : Inport
  FB : Inport  Port=2
  Add : Sum
  Bus Selector3 : BusSelector  OutputSignals=torque
  FB Torque : Outport
  wires:
  Bus Selector3/1 -> Add/1  "<torque>"
  FB/1 -> Add/2
  Add/1 -> FB Torque/1
  Torque/1 -> Bus Selector3/1

== system VCM_main/VDC/80kw_limitation/Power Limit_last/FeedBack2 ==
  Torque : Inport
  FB : Inport  Port=2
  Add : Sum
  Bus Selector3 : BusSelector  OutputSignals=torque
  FB Torque : Outport
  wires:
  Torque/1 -> Bus Selector3/1
  Add/1 -> FB Torque/1
  FB/1 -> Add/2
  Bus Selector3/1 -> Add/1  "<torque>"

== system VCM_main/VDC/80kw_limitation/Power Limit_last/FeedBack3 ==
  Torque : Inport
  FB : Inport  Port=2
  Add : Sum
  Bus Selector3 : BusSelector  OutputSignals=torque
  FB Torque : Outport
  wires:
  Bus Selector3/1 -> Add/1  "<torque>"
  FB/1 -> Add/2
  Add/1 -> FB Torque/1
  Torque/1 -> Bus Selector3/1

== system VCM_main/VDC/DYC1/DYC main/DYC ecopa spec ==
  Total Torque In : Inport
  DriverInput : Inport  Port=2
  Sensor : Inport  Port=3
  Action Port : ActionPort
  DYC mode2 : Subsystem
  DYC_K : Outport
  DYC_M : Outport  Port=2
  DYC_RR : Outport  Port=3
  DYC_RL : Outport  Port=4
  DYC_FR : Outport  Port=5
  DYC_FL : Outport  Port=6
  wires:
  DYC mode2/6(DYC_FL) -> DYC_FL/1
  DYC mode2/5(DYC_FR) -> DYC_FR/1
  DYC mode2/4(DYC_RL) -> DYC_RL/1
  DYC mode2/3(DYC_RR) -> DYC_RR/1
  DYC mode2/2(DYC_M) -> DYC_M/1  "Moment"
  Sensor/1 -> DYC mode2/3(Sensor)
  DriverInput/1 -> DYC mode2/2(DriverInput)
  DYC mode2/1(DYC_K) -> DYC_K/1  "Gain"
  Total Torque In/1 -> DYC mode2/1(Total Torque In)

== system VCM_main/VDC/DYC1/DYC main/DYC mode1 ==
  Total Torque In : Inport
  DriverInput : Inport  Port=2
  Sensor : Inport  Port=3
  from_steerSW : Inport  Port=4
  Action Port : ActionPort
  DYC mode1 : Subsystem
  DYC_K : Outport
  DYC_M : Outport  Port=2
  DYC_RR : Outport  Port=3
  DYC_RL : Outport  Port=4
  DYC_FR : Outport  Port=5
  DYC_FL : Outport  Port=6
  wires:
  from_steerSW/1 -> DYC mode1/4(from_steerswitch)
  DYC mode1/6(DYC_FL) -> DYC_FL/1
  DYC mode1/5(DYC_FR) -> DYC_FR/1
  DYC mode1/4(DYC_RL) -> DYC_RL/1
  DYC mode1/3(DYC_RR) -> DYC_RR/1
  DYC mode1/2(DYC_M) -> DYC_M/1  "Moment"
  Sensor/1 -> DYC mode1/3(Sensor)
  DriverInput/1 -> DYC mode1/2(DriverInput)
  DYC mode1/1(DYC_K) -> DYC_K/1  "Gain"
  Total Torque In/1 -> DYC mode1/1(Total Torque In)

== system VCM_main/VDC/Traction Control/Fx Estimater/FxEstimater ==
  Torque : Inport
  ActualSpeed : Inport  Port=2
  Add4 : Sum  Inputs=+-
  Discrete Derivative : simulink/Discrete/Discrete Derivative  gainval=1.0  ICPrevScaledInput=0.0  OutMin=[]  OutMax=[]  OutDataType=fixdt(1, 16)  OutScaling=2^-10  DoSatur=off
  Gain : Gain  Gain=gear_f
  Gain1 : Gain  Gain=1/60
  Gain2 : Gain  Gain=2*pi
  Gain3 : Gain  Gain=1/gear_f
  Gain4 : Gain  Gain=Iwf
  Gain5 : Gain  Gain=1/Rwf
  Fx : Outport
  wires:
  Gain1/1 -> Gain2/1
  Gain2/1 -> Discrete Derivative/1
  Torque/1 -> Gain/1
  Discrete Derivative/1 -> Gain4/1
  Gain/1 -> Add4/1
  Add4/1 -> Gain5/1
  Gain5/1 -> Fx/1
  Gain4/1 -> Add4/2
  ActualSpeed/1 -> Gain3/1
  Gain3/1 -> Gain1/1

== system VCM_main/VDC/Traction Control/Fx Estimater/FxEstimater1 ==
  Torque : Inport
  ActualSpeed : Inport  Port=2
  Add4 : Sum  Inputs=+-
  Discrete Derivative : simulink/Discrete/Discrete Derivative  gainval=1.0  ICPrevScaledInput=0.0  OutMin=[]  OutMax=[]  OutDataType=fixdt(1, 16)  OutScaling=2^-10  DoSatur=off
  Gain : Gain  Gain=gear_f
  Gain1 : Gain  Gain=1/60
  Gain2 : Gain  Gain=2*pi
  Gain3 : Gain  Gain=1/gear_f
  Gain4 : Gain  Gain=Iwf
  Gain5 : Gain  Gain=1/Rwf
  Fx : Outport
  wires:
  Gain3/1 -> Gain1/1
  ActualSpeed/1 -> Gain3/1
  Gain4/1 -> Add4/2
  Gain5/1 -> Fx/1
  Add4/1 -> Gain5/1
  Gain/1 -> Add4/1
  Discrete Derivative/1 -> Gain4/1
  Torque/1 -> Gain/1
  Gain2/1 -> Discrete Derivative/1
  Gain1/1 -> Gain2/1

== system VCM_main/VDC/Traction Control/Fx Estimater/FxEstimater2 ==
  Torque : Inport
  ActualSpeed : Inport  Port=2
  Add4 : Sum  Inputs=+-
  Discrete Derivative : simulink/Discrete/Discrete Derivative  gainval=1.0  ICPrevScaledInput=0.0  OutMin=[]  OutMax=[]  OutDataType=fixdt(1, 16)  OutScaling=2^-10  DoSatur=off
  Gain : Gain  Gain=gear_f
  Gain1 : Gain  Gain=1/60
  Gain2 : Gain  Gain=2*pi
  Gain3 : Gain  Gain=1/gear_f
  Gain4 : Gain  Gain=Iwf
  Gain5 : Gain  Gain=1/Rwf
  Fx : Outport
  wires:
  Gain1/1 -> Gain2/1
  Gain2/1 -> Discrete Derivative/1
  Torque/1 -> Gain/1
  Discrete Derivative/1 -> Gain4/1
  Gain/1 -> Add4/1
  Add4/1 -> Gain5/1
  Gain5/1 -> Fx/1
  Gain4/1 -> Add4/2
  ActualSpeed/1 -> Gain3/1
  Gain3/1 -> Gain1/1

== system VCM_main/VDC/Traction Control/Fx Estimater/FxEstimater3 ==
  Torque : Inport
  ActualSpeed : Inport  Port=2
  Add4 : Sum  Inputs=+-
  Discrete Derivative : simulink/Discrete/Discrete Derivative  gainval=1.0  ICPrevScaledInput=0.0  OutMin=[]  OutMax=[]  OutDataType=fixdt(1, 16)  OutScaling=2^-10  DoSatur=off
  Gain : Gain  Gain=gear_f
  Gain1 : Gain  Gain=1/60
  Gain2 : Gain  Gain=2*pi
  Gain3 : Gain  Gain=1/gear_f
  Gain4 : Gain  Gain=Iwf
  Gain5 : Gain  Gain=1/Rwf
  Fx : Outport
  wires:
  Gain3/1 -> Gain1/1
  ActualSpeed/1 -> Gain3/1
  Gain4/1 -> Add4/2
  Gain5/1 -> Fx/1
  Add4/1 -> Gain5/1
  Gain/1 -> Add4/1
  Discrete Derivative/1 -> Gain4/1
  Torque/1 -> Gain/1
  Gain2/1 -> Discrete Derivative/1
  Gain1/1 -> Gain2/1

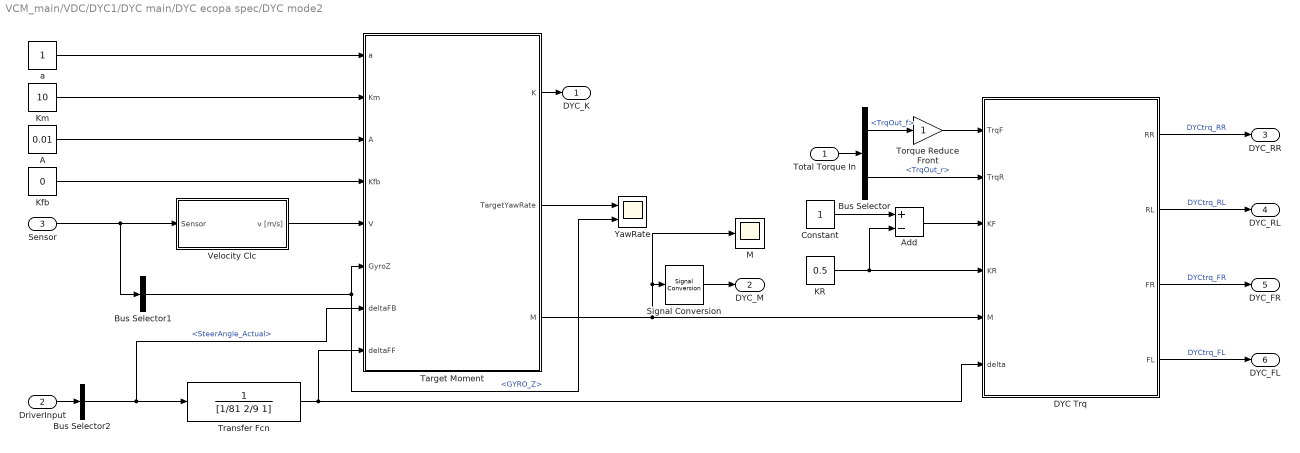
== system VCM_main/VDC/DYC1/DYC main/DYC ecopa spec/DYC mode2 ==
  Total Torque In : Inport
  DriverInput : Inport  Port=2
  Sensor : Inport  Port=3
  A : Constant  Value=0.01
  Add : Sum  Inputs=+-
  Bus Selector : BusSelector  OutputSignals=TrqOut_f,TrqOut_r
  Bus Selector1 : BusSelector  OutputSignals=CAN_from_IMU_122.GYRO_Z
  Bus Selector2 : BusSelector  OutputSignals=SteerAngle_Actual
  Constant : Constant
  DYC Trq : MATLAB Function  TreatAsAtomicUnit=on
  KR : Constant  Value=0.5
  Kfb : Constant  Value=0
  Km : Constant  Value=10
  M : Scope
  Signal Conversion : SignalConversion  OverrideOpt=off
  Target Moment : MATLAB Function  TreatAsAtomicUnit=on
  Torque Reduce Front : Gain
  Transfer Fcn : TransferFcn  Denominator=[1/81 2/9 1]
  Velocity Clc : Subsystem
  YawRate : Scope  NumInputPorts=2
  a : Constant
  DYC_K : Outport
  DYC_M : Outport  Port=2
  DYC_RR : Outport  Port=3
  DYC_RL : Outport  Port=4
  DYC_FR : Outport  Port=5
  DYC_FL : Outport  Port=6
  wires:
  Signal Conversion/1 -> DYC_M/1
  Torque Reduce Front/1 -> DYC Trq/1(TrqF)
  Target Moment/2(TargetYawRate) -> YawRate/1
  Target Moment/3(M) -> DYC Trq/5(M), M/1, Signal Conversion/1
  A/1 -> Target Moment/3(A)
  Bus Selector1/1 -> YawRate/2, Target Moment/6(GyroZ)  "<GYRO_Z>"
  Sensor/1 -> Velocity Clc/1(Sensor), Bus Selector1/1
  a/1 -> Target Moment/1(a)
  Transfer Fcn/1 -> DYC Trq/6(delta), Target Moment/8(deltaFF)
  DYC Trq/4(FL) -> DYC_FL/1  "DYCtrq_FL"
  DYC Trq/3(FR) -> DYC_FR/1  "DYCtrq_FR"
  DYC Trq/2(RL) -> DYC_RL/1  "DYCtrq_RL"
  DYC Trq/1(RR) -> DYC_RR/1  "DYCtrq_RR"
  Constant/1 -> Add/1
  KR/1 -> DYC Trq/4(KR), Add/2
  Add/1 -> DYC Trq/3(KF)
  Bus Selector/2 -> DYC Trq/2(TrqR)  "<TrqOut_r>"
  Bus Selector/1 -> Torque Reduce Front/1  "<TrqOut_f>"
  Total Torque In/1 -> Bus Selector/1
  Bus Selector2/1 -> Transfer Fcn/1, Target Moment/7(deltaFB)  "<SteerAngle_Actual>"
  Kfb/1 -> Target Moment/4(Kfb)
  Km/1 -> Target Moment/2(Km)
  Velocity Clc/1(v [m/s]) -> Target Moment/5(V)
  DriverInput/1 -> Bus Selector2/1
  Target Moment/1(K) -> DYC_K/1

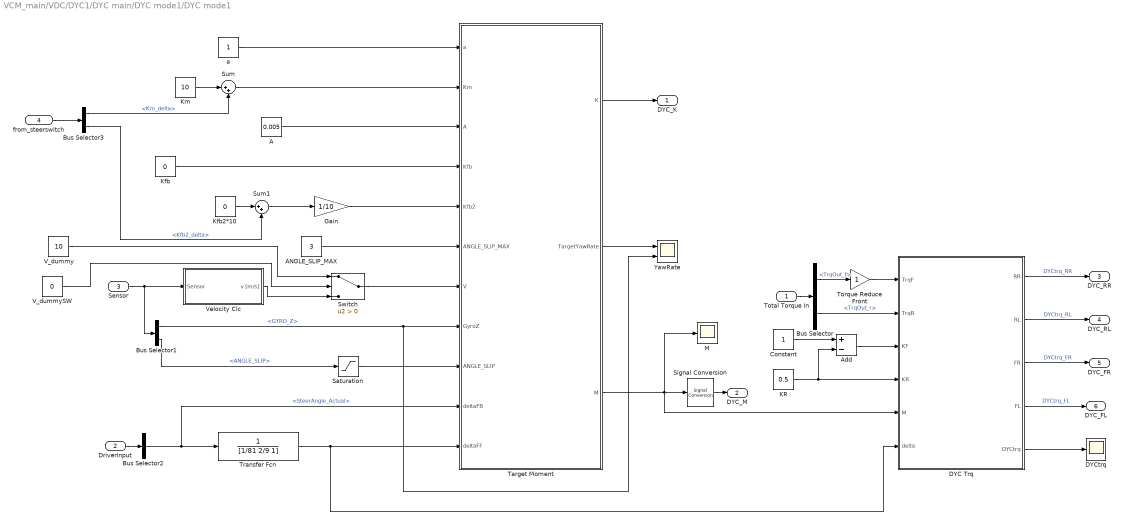
== system VCM_main/VDC/DYC1/DYC main/DYC mode1/DYC mode1 ==
  Total Torque In : Inport
  DriverInput : Inport  Port=2
  Sensor : Inport  Port=3
  from_steerswitch : Inport  Port=4
  A : Constant  Value=0.005
  ANGLE_SLIP_MAX : Constant  Value=3
  Add : Sum  Inputs=+-
  Bus Selector : BusSelector  OutputSignals=TrqOut_f,TrqOut_r
  Bus Selector1 : BusSelector  OutputSignals=CAN_from_IMU_122.GYRO_Z,CAN_from_IMU_220.ANGLE_SLIP
  Bus Selector2 : BusSelector  OutputSignals=SteerAngle_Actual
  Bus Selector3 : BusSelector  OutputSignals=Km_delta,Kfb2_delta
  Constant : Constant
  DYC Trq : MATLAB Function  TreatAsAtomicUnit=on
  DYCtrq : Scope
  Gain : Gain  Gain=1/10
  KR : Constant  Value=0.5
  Kfb : Constant  Value=0
  Kfb2*10 : Constant  Value=0
  Km : Constant  Value=10
  M : Scope
  Saturation : Saturate  UpperLimit=20  LowerLimit=-20
  Signal Conversion : SignalConversion  OverrideOpt=off
  Sum : Sum  Inputs=|++
  Sum1 : Sum  Inputs=|++
  Switch : Switch  Criteria=u2 > Threshold
  Target Moment : MATLAB Function  TreatAsAtomicUnit=on
  Torque Reduce Front : Gain
  Transfer Fcn : TransferFcn  Denominator=[1/81 2/9 1]
  V_dummy : Constant  Value=10
  V_dummySW : Constant  Value=0
  Velocity Clc : Subsystem
  YawRate : Scope  NumInputPorts=2
  a : Constant
  DYC_K : Outport
  DYC_M : Outport  Port=2
  DYC_RR : Outport  Port=3
  DYC_RL : Outport  Port=4
  DYC_FR : Outport  Port=5
  DYC_FL : Outport  Port=6
  wires:
  V_dummySW/1 -> Switch/2
  V_dummy/1 -> Switch/1
  Switch/1 -> Target Moment/7(V)
  Gain/1 -> Target Moment/5(Kfb2)
  Saturation/1 -> Target Moment/9(ANGLE_SLIP)
  DYC Trq/5(DYCtrq) -> DYCtrq/1
  Bus Selector3/1 -> Sum/2  "<Km_delta>"
  from_steerswitch/1 -> Bus Selector3/1
  Signal Conversion/1 -> DYC_M/1
  ANGLE_SLIP_MAX/1 -> Target Moment/6(ANGLE_SLIP_MAX)
  Bus Selector1/2 -> Saturation/1  "<ANGLE_SLIP>"
  Bus Selector3/2 -> Sum1/2  "<Kfb2_delta>"
  Kfb2*10/1 -> Sum1/1
  Sum1/1 -> Gain/1
  Km/1 -> Sum/1
  Torque Reduce Front/1 -> DYC Trq/1(TrqF)
  Target Moment/2(TargetYawRate) -> YawRate/1
  Target Moment/3(M) -> DYC Trq/5(M), Signal Conversion/1, M/1
  A/1 -> Target Moment/3(A)
  Bus Selector1/1 -> YawRate/2, Target Moment/8(GyroZ)  "<GYRO_Z>"
  Sensor/1 -> Velocity Clc/1(Sensor), Bus Selector1/1
  a/1 -> Target Moment/1(a)
  Transfer Fcn/1 -> DYC Trq/6(delta), Target Moment/11(deltaFF)
  DYC Trq/4(FL) -> DYC_FL/1  "DYCtrq_FL"
  DYC Trq/3(FR) -> DYC_FR/1  "DYCtrq_FR"
  DYC Trq/2(RL) -> DYC_RL/1  "DYCtrq_RL"
  DYC Trq/1(RR) -> DYC_RR/1  "DYCtrq_RR"
  Constant/1 -> Add/1
  KR/1 -> DYC Trq/4(KR), Add/2
  Add/1 -> DYC Trq/3(KF)
  Bus Selector/2 -> DYC Trq/2(TrqR)  "<TrqOut_r>"
  Bus Selector/1 -> Torque Reduce Front/1  "<TrqOut_f>"
  Total Torque In/1 -> Bus Selector/1
  Bus Selector2/1 -> Transfer Fcn/1, Target Moment/10(deltaFB)  "<SteerAngle_Actual>"
  Kfb/1 -> Target Moment/4(Kfb)
  Sum/1 -> Target Moment/2(Km)
  Velocity Clc/1(v [m/s]) -> Switch/3
  DriverInput/1 -> Bus Selector2/1
  Target Moment/1(K) -> DYC_K/1

== system VCM_main/VDC/DYC1/DYC main/DYC ecopa spec/DYC mode2/Velocity Clc ==
  Sensor : Inport
  Add : Sum
  Bus Selector : BusSelector  OutputSignals=CAN_from_IMU_139.VELOCITY_X,CAN_from_IMU_139.VELOCITY_Y
  Sqrt : Sqrt  SaturateOnIntegerOverflow=on
  Square1 : Math  Operator=square  SaturateOnIntegerOverflow=on
  Square2 : Math  Operator=square  SaturateOnIntegerOverflow=on
  Transfer Fcn : TransferFcn  Denominator=[0.03 1]
  v [m/s] : Outport
  wires:
  Sqrt/1 -> Transfer Fcn/1  "v [m/s]"
  Transfer Fcn/1 -> v [m/s]/1  "v [m/s]"
  Square2/1 -> Add/2
  Sensor/1 -> Bus Selector/1
  Square1/1 -> Add/1
  Add/1 -> Sqrt/1
  Bus Selector/1 -> Square1/1  "<VELOCITY_X>"
  Bus Selector/2 -> Square2/1  "<VELOCITY_Y>"

== system VCM_main/VDC/DYC1/DYC main/DYC mode1/DYC mode1/Velocity Clc ==
  Sensor : Inport
  Add : Sum
  Bus Selector : BusSelector  OutputSignals=CAN_from_IMU_139.VELOCITY_X,CAN_from_IMU_139.VELOCITY_Y
  Sqrt : Sqrt  SaturateOnIntegerOverflow=on
  Square1 : Math  Operator=square  SaturateOnIntegerOverflow=on
  Square2 : Math  Operator=square  SaturateOnIntegerOverflow=on
  Transfer Fcn : TransferFcn  Denominator=[0.03 1]
  v [m/s] : Outport
  wires:
  Sqrt/1 -> Transfer Fcn/1  "v [m/s]"
  Transfer Fcn/1 -> v [m/s]/1  "v [m/s]"
  Square2/1 -> Add/2
  Sensor/1 -> Bus Selector/1
  Square1/1 -> Add/1
  Add/1 -> Sqrt/1
  Bus Selector/1 -> Square1/1  "<VELOCITY_X>"
  Bus Selector/2 -> Square2/1  "<VELOCITY_Y>"

== matlab function VCM_main/VDC/DYC1/DYC main/DYC mode1/DYC mode1/Target Moment ==
  data: a input; Km input; A input; Kfb input; Kfb2 input; ANGLE_SLIP_MAX input; K output; TargetYawRate output; V input; GyroZ input; ANGLE_SLIP input; deltaFB input; deltaFF input; M output; l parameter
function [K, TargetYawRate, M] = fcn(a, Km, A, Kfb, Kfb2, ANGLE_SLIP_MAX, V, GyroZ, ANGLE_SLIP, deltaFB, deltaFF, l)
    if V<3/3.6
        K=0;
        TargetYawRate=0;
        M=0;
    else
        x0=(Km/2/a + 40)/3.6;
        K=Km*(1/(1+exp(a*(V-x0))));
        Kfb=Kfb*(1/(1+exp(a*(V-x0))));
        TargetYawRate=(1/(1+A*V*V))*(V/l)*deltaFB;
        M=K*deltaFF+Kfb*(TargetYawRate-GyroZ);
        if GyroZ > 0
            if ANGLE_SLIP > ANGLE_SLIP_MAX
                M=M-Kfb2(ANGLE_SLIP-ANGLE_SLIP_MAX);
            end
        else
            if -ANGLE_SLIP > ANGLE_SLIP_MAX
                M=M+Kfb2(-ANGLE_SLIP-ANGLE_SLIP_MAX);
            end
        end
    end
end
